simulink model "prob1"  (R2019a)
settings: Solver=VariableStepAuto  StartTime=0.0  StopTime=10.0  RelTol=1e-3
values from neighbouring files (symbols this model uses):
  bias = 1E-3 * g    (= 0.0097803267714)    [prob1main.m]
  delH0 = 0    [prob1main.m]
  delV0 = 0    [prob1main.m]
  g = 9.7803267714    [prob1main.m]
  noise = 0    [prob1main.m]
  R = 6378137    [prob1main.m]
settings Model: Creator=hyunwoong  LastModifiedBy=hyunwoong

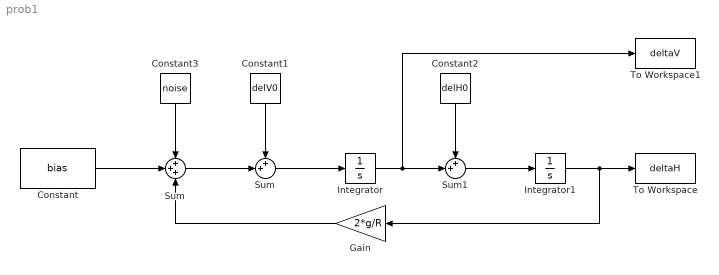
== system prob1 ==
  Constant : Constant  Value=bias
  Constant1 : Constant  Value=delV0
  Constant2 : Constant  Value=delH0
  Constant3 : Constant  Value=noise
  Gain : Gain  Gain=2*g/R
  Integrator : Integrator
  Integrator1 : Integrator
  Sum : Sum  Inputs=++|
  "Sum " : Sum  Inputs=+++
  Sum1 : Sum  Inputs=++|
  To Workspace : ToWorkspace  VariableName=deltaH  SaveFormat=Timeseries  SampleTime=-1
  To Workspace1 : ToWorkspace  VariableName=deltaV  SaveFormat=Timeseries  SampleTime=-1
  wires:
  Constant/1 -> "Sum "/2
  "Sum "/1 -> Sum/2
  Integrator/1 -> To Workspace1/1, Sum1/2
  Sum/1 -> Integrator/1
  Constant1/1 -> Sum/1
  Constant2/1 -> Sum1/1
  Integrator1/1 -> Gain/1, To Workspace/1
  Sum1/1 -> Integrator1/1
  Constant3/1 -> "Sum "/1
  Gain/1 -> "Sum "/3
